simulink model "DAQsl_12lead_SZ_v3"  (R2014a)
settings: Solver=FixedStepDiscrete  StartTime=0.0  StopTime=Inf  RelTol=1e-3
undefined symbols (not defined in the file): analoginput
libraries: dspsigops x3, dspindex x3, daqlib x1
settings Model: Creator=Ssubrama  LastModifiedBy=xw8600
settings DataIOCC: MaxDataPoints=10000  SaveOutput=off  SaveTime=off
settings OptimizationCC: InitFltsAndDblsToZero=on
settings DebuggingCC: SaveWithParameterizedLinksMsg=none  UnderspecifiedInitializationDetection=Classic  SignalResolutionControl=TryResolveAllWithWarning  FcnCallInpInsideContextMsg=UseLocalSettings
settings HardwareCC: ProdBitPerLong=64  ProdBitPerPointer=64  ProdIntDivRoundTo=Zero  ProdEndianess=LittleEndian  ProdWordSize=64  ProdHWDeviceType=Intel->x86-64
settings GRTTargetCC: TargetFcnLib=ansi_tfl_tmw.mat  CombineOutputUpdateFcns=off  GRTInterface=on

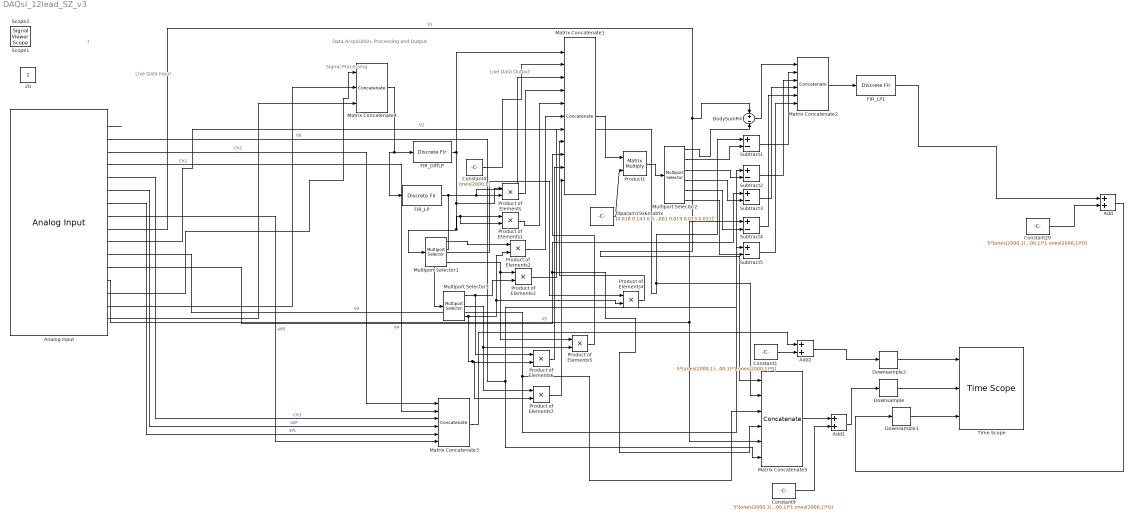
== system DAQsl_12lead_SZ_v3 ==
  note: Live Data Input
  note: Signal Processing
  note: Live Data Output
  note: ?
  note: Data Acquisition, Processing and Output
  Add : Sum
  Add1 : Sum
  Add2 : Sum
  Analog Input : daqlib/Analog Input  AcqMode=0  DeviceMenu=nidaq Dev3 (PCI-6251)  Device=nidaq Dev3 (PCI-6251)  ObjConstructor=analoginput('nidaq','Dev3')  SampleRate=48000  ActualRate=48076.9231  SamplesPerFrame=2000  InputType=SingleEnded  NChannelsSelected=16  Channels=1$0$TTL$1$#1$1$V6$1$#1$2$Ch1$1$#1$3$Ch2$1$#1$4$Ch3$1$#1$5$aVF$1$#1$6$aVL$1$#1$7$aVR$1$#1$8$V1$1$#1$9$V2$1$#1$10$V3$1$#1$11$V4$1$#1$12$V5$1$#1$13$Gx$1$#1$14$Gy$1$#1$15$Gz$1$#  NPorts=1 per hardware channel  DataType=double
      settings: SignalType=Frame-based
  BodySumR4 : Sum  Inputs=+-  SaturateOnIntegerOverflow=on  InputSameDT=on  OutDataTypeStr=Inherit: Same as first input
  Constant1 : Constant  Value=5*[ones(2000,1)*5 ones(2000,1)*4 ones(2000,1)*3 ones(2000,1)*2 ones(2000,1)*1 ones(2000,1)*0]  VectorParams1D=off
      settings: SamplingMode=Frame based
  Constant20 : Constant  Value=5*[ones(2000,1)*5 ones(2000,1)*4 ones(2000,1)*3 ones(2000,1)*2 ones(2000,1)*1 ones(2000,1)*0]  VectorParams1D=off
      settings: SamplingMode=Frame based
  Constant4 : Constant  Value=ones(2000,1)
  Constant9 : Constant  Value=5*[ones(2000,1)*5 ones(2000,1)*4 ones(2000,1)*3 ones(2000,1)*2 ones(2000,1)*1 ones(2000,1)*0]  VectorParams1D=off
      settings: SamplingMode=Frame based
  Downsample : dspsigops/Downsample  N=20  phase=0  InputProcessing=Columns as channels (frame based)  RateOptions=Enforce single-rate processing  smode=Allow multirate  fmode=Maintain input frame size  ic=0
  Downsample1 : dspsigops/Downsample  N=20  phase=0  InputProcessing=Columns as channels (frame based)  RateOptions=Enforce single-rate processing  smode=Allow multirate  fmode=Maintain input frame size  ic=0
  Downsample2 : dspsigops/Downsample  N=20  phase=0  InputProcessing=Columns as channels (frame based)  RateOptions=Enforce single-rate processing  smode=Allow multirate  fmode=Maintain input frame size  ic=0
  FIR_DiffLP : DiscreteFir  Tag=BlockMethodSubSystem  Coefficients=[-0.18062676936828148 0.075498218012372678 0.060163267428857255 0.047127582079132126 0.036106819784294142 0.02681014925394444 0.019028739148422402 0.012533880333517169 0.0071669984796646352 0.0027552314840064152 -0.00081448231664470183 -0.0036806791908466363 -0.0059307473989848453 -0.0076730993176787332 -0.0089619539864591313 -0.0098834705132522516 -0.010476162627155713 -0.010815439651932726 -0.010922412979674896 -0.010854092940204011 -0.010623964947882394 -0.010281828260079147 -0.0098295768735839738 -0.0093076194808661503 -0.0087171332221934409 -0.0080952195518808889 -0.0074299916490935501 -0.0067566400598708665 -0.0060669163247976596 -0.0053840878831306546 -0.0046956715284624667 -0.0040267199297590664 -0.0033675351882764826 -0.0027286000751785278 -0.002108607617879607 -0.0015238417303873875 -0.00094743192210984539 -0.00041768033371966662 9.7957895782735394e-05 0.00057601238716023517 0.0010248307888518354 0.0014437654277015821 0.0018365593501642741 0.0021923858617342723 0.0025292384839017273 0.0028281832383850597 0.0031059437646882987 0.0033443496347939569 0.0035673730523742425 0.003752427774854239 0.0039229917726955055 0.0040619759986883358 0.0041874782442662406 0.0042782756027622271 0.0043576942897668378 0.0044067060750872349 0.0044457562817536884 0.0044540410288122848 0.0044560643720905277 0.0044305989660153788 0.0043983184651787306 0.0043414367775261621 0.0042806358872290026 0.0041964625041126316 0.0041077120934579527 0.0039952274460846749 0.0038828867568738781 0.0037512724746293011 0.0036205033327657669 0.0034736791748717216 0.0032889244822337099 0.0032254429105413249 0.0028652076907176929 0.0029082850211105266 0.0026479711649063722 0.0023587308162685075 0.0022528173108101665 0.0021190210876191606 0.0018837093920242853 0.0016159764478156438 0.0014255307135332407 0.0012722914566817081 0.0011051792687347683 0.00087391216090881851 0.00062790988577039741 0.0003947553207023502 0.00021307525542524353 3.8419429882835532e-05 -0.00013851866134199919 -0.00035331824585213556 -0.00057153746455100574 -0.00079518720639934481 -0.00099088393330477864 -0.0011768847795266338 -0.0013366611902774078 -0.0015049172753172635 -0.0016743468203979442 -0.0018681775384048055 -0.0020506287994834366 -0.0022350623124652511 -0.0023958814720651395 -0.0025455246897644196 -0.0026681493794683125 -0.0027953157186838759 -0.0029185414486199504 -0.0030470602313935821 -0.003170822638784352 -0.0033062616061319827 -0.0034083685540330644 -0.0035137506831716507 -0.0035917717472638555 -0.0036552967807502047 -0.0037115002611477748 -0.0037592929285841514 -0.0038012849278920291 -0.0038484314440238665 -0.0038809552016502939 -0.003915923816400658 -0.0039318204175490864 -0.0039468513375555975 -0.0039355527248360334 -0.0039219335995399861 -0.0038850405920592482 -0.0038456166297130279 -0.0037875584268758089 -0.0037357892367000725 -0.0036680486958331343 -0.0036056218772497206 -0.0035256875435648108 -0.0034475962249451778 -0.0033445595331721492 -0.0032391637968775672 -0.0031120075764690808 -0.0029828631931814453 -0.0028318144386076383 -0.0026811043906390386 -0.0025110952371861922 -0.0023453505568085814 -0.002163846592305646 -0.0019895103237992234 -0.001801291958943102 -0.0016072154014195456 -0.0014196945636693326 -0.0011730884740853986 -0.00099911632268769035 -0.00073404218139398736 -0.00049829192144557055 -0.00028549369653109447 -5.506282783576677e-06 0.00024919397633001161 0.00048353320834738922 0.00072833962518251139 0.0010114071500255395 0.0012749539678287153 0.0015276715389412471 0.0017769189385540562 0.0020582940564560365 0.0023362045534717768 0.002614202508477409 0.0028710136230506861 0.0031473512240854928 0.0034284462133270521 0.0037253606974353981 0.0039994098214293505 0.0042699259854619004 0.0045289443247042843 0.0048076546226093128 0.0050751764458327117 0.0053398886724922226 0.0055788878033309307 0.0058266068769547291 0.0060625331374312072 0.0063039444342566746 0.006536104937273835 0.0067761788261536636 0.0069916195956320716 0.0071980099546128367 ...(+6580 chars)]  InputProcessing=Columns as channels (frame based)
  FIR_LP : DiscreteFir  Tag=BlockMethodSubSystem  Coefficients=[-0.016046831360515792 -0.00065949202963794772 -0.00067039658894896444 -0.000680113961541811 -0.00068755840268027585 -0.00069373348662863862 -0.00069825998158766847 -0.00070062225893785003 -0.00070116943134638197 -0.00069998300862922705 -0.00069683650818794934 -0.00069174377031850157 -0.00068465891805698231 -0.0006754671176039586 -0.00066426308006034725 -0.00065111557687173513 -0.00063595716866335708 -0.00061876858965746219 -0.00059952370199125617 -0.00057816905133744462 -0.00055474993594159874 -0.00052933462980164249 -0.00050193501018345847 -0.00047257449533386758 -0.00044127300464813848 -0.00040802895812505624 -0.00037287875518891844 -0.00033587281713210425 -0.00029703591839722911 -0.00025639926655389098 -0.00021400511216308066 -0.000169903979016367 -0.00012417368617071919 -7.6899072060668261e-05 -2.8150157008115934e-05 2.2012840404119632e-05 7.3532898375517491e-05 0.00012633250117251651 0.00018030739853822954 0.00023534639937773834 0.00029132592147520543 0.00034812020483494278 0.00040561154772518829 0.00046364631505794313 0.00052204804071215652 0.00058066809893052296 0.00063935345308781776 0.00069795947359434403 0.00075638331683252659 0.0008144673153936393 0.00087200667052411175 0.00092886523071337816 0.00098491103491506193 0.0010400300146259991 0.0010942443343466991 0.0011475182049489208 0.0011996969814079186 0.0012507656741247899 0.0013006677104798262 0.0013491930666350918 0.0013963602484677647 0.0014419368978449854 0.0014849360919130389 0.0015246732347401933 0.0015604329877536675 0.001589663683854995 0.0016110689442300034 0.0016626488924509492 0.0016801670749969633 0.0017034055881406177 0.0017242062257781157 0.001740884608416331 0.0017545721087722163 0.0017652528489535933 0.0017721296593393495 0.0017752870822966265 0.001774898562581546 0.001770787995046345 0.001762960472003177 0.0017513748993286012 0.0017357956194428426 0.0017161802261388345 0.0016926022018635637 0.0016650502257861671 0.0016335578945971853 0.0015981504382308574 0.0015587555258380591 0.0015153562862723416 0.0014680048047343904 0.00141673289877608 0.0013616004323335849 0.0013026840428024839 0.0012400261833809371 0.0011736954590057282 0.0011037979083276649 0.0010304273240276402 0.00095367644473309983 0.00087363714813433989 0.00079039072069638991 0.00070404458701325487 0.00061474337339734522 0.00052265102521284468 0.00042794153165760102 0.00033078244735946713 0.00023134271266805548 0.00012981038374990442 2.6383866326591676e-05 -7.8720638387243247e-05 -0.0001852791260239621 -0.00029309255066418093 -0.00040194826579460254 -0.00051159688026453619 -0.00062179525337211113 -0.00073228421262779182 -0.00084280009755509887 -0.00095315646127709479 -0.0010631698123428675 -0.0011725907339674574 -0.0012811859886916917 -0.0013886724649219331 -0.0014946824753083818 -0.0015989506657064674 -0.0017012114004422568 -0.0018010383222902843 -0.0018981003457104201 -0.0019921033209773596 -0.0020826208663505107 -0.0021696373876007296 -0.0022534152697132274 -0.0023336529410050173 -0.0024101808555453772 -0.0024829460735073614 -0.0025493465368724936 -0.0026056342923423959 -0.0026660896237801039 -0.0027155873088072248 -0.0027597560898392805 -0.0027992138857687344 -0.0028312885749167023 -0.0028568226553243887 -0.0028762651224427203 -0.0028887281907468195 -0.0028938572083181211 -0.0028916490204876754 -0.0028818357929839816 -0.0028643621005438689 -0.0028392507802816064 -0.0028062271598547107 -0.0027650433892605526 -0.0027155849769926309 -0.0026576966095576051 -0.0025913119936476301 -0.002516447996338678 -0.0024330280889569983 -0.002340965996042766 -0.0022402306543335519 -0.0021307704474492657 -0.0020125592717875045 -0.0018856146073182398 -0.0017499232285739519 -0.0016054780056661694 -0.0014523244548257722 -0.001290529994776534 -0.001120190883235693 -0.00094142800833800153 -0.00075434593435997482 -0.00055904539805591569 -0.00035564822940898841 -0.00014430020616271189 7.4822152403616199e-05 0.00030152760804075251 0.00053562169595984185 0.00077689558294914522 0.0010251305942399983 ...(+6591 chars)]  InputProcessing=Columns as channels (frame based)
  FIR_LP1 : DiscreteFir  Tag=BlockMethodSubSystem  Coefficients=[-0.016046831360515792 -0.00065949202963794772 -0.00067039658894896444 -0.000680113961541811 -0.00068755840268027585 -0.00069373348662863862 -0.00069825998158766847 -0.00070062225893785003 -0.00070116943134638197 -0.00069998300862922705 -0.00069683650818794934 -0.00069174377031850157 -0.00068465891805698231 -0.0006754671176039586 -0.00066426308006034725 -0.00065111557687173513 -0.00063595716866335708 -0.00061876858965746219 -0.00059952370199125617 -0.00057816905133744462 -0.00055474993594159874 -0.00052933462980164249 -0.00050193501018345847 -0.00047257449533386758 -0.00044127300464813848 -0.00040802895812505624 -0.00037287875518891844 -0.00033587281713210425 -0.00029703591839722911 -0.00025639926655389098 -0.00021400511216308066 -0.000169903979016367 -0.00012417368617071919 -7.6899072060668261e-05 -2.8150157008115934e-05 2.2012840404119632e-05 7.3532898375517491e-05 0.00012633250117251651 0.00018030739853822954 0.00023534639937773834 0.00029132592147520543 0.00034812020483494278 0.00040561154772518829 0.00046364631505794313 0.00052204804071215652 0.00058066809893052296 0.00063935345308781776 0.00069795947359434403 0.00075638331683252659 0.0008144673153936393 0.00087200667052411175 0.00092886523071337816 0.00098491103491506193 0.0010400300146259991 0.0010942443343466991 0.0011475182049489208 0.0011996969814079186 0.0012507656741247899 0.0013006677104798262 0.0013491930666350918 0.0013963602484677647 0.0014419368978449854 0.0014849360919130389 0.0015246732347401933 0.0015604329877536675 0.001589663683854995 0.0016110689442300034 0.0016626488924509492 0.0016801670749969633 0.0017034055881406177 0.0017242062257781157 0.001740884608416331 0.0017545721087722163 0.0017652528489535933 0.0017721296593393495 0.0017752870822966265 0.001774898562581546 0.001770787995046345 0.001762960472003177 0.0017513748993286012 0.0017357956194428426 0.0017161802261388345 0.0016926022018635637 0.0016650502257861671 0.0016335578945971853 0.0015981504382308574 0.0015587555258380591 0.0015153562862723416 0.0014680048047343904 0.00141673289877608 0.0013616004323335849 0.0013026840428024839 0.0012400261833809371 0.0011736954590057282 0.0011037979083276649 0.0010304273240276402 0.00095367644473309983 0.00087363714813433989 0.00079039072069638991 0.00070404458701325487 0.00061474337339734522 0.00052265102521284468 0.00042794153165760102 0.00033078244735946713 0.00023134271266805548 0.00012981038374990442 2.6383866326591676e-05 -7.8720638387243247e-05 -0.0001852791260239621 -0.00029309255066418093 -0.00040194826579460254 -0.00051159688026453619 -0.00062179525337211113 -0.00073228421262779182 -0.00084280009755509887 -0.00095315646127709479 -0.0010631698123428675 -0.0011725907339674574 -0.0012811859886916917 -0.0013886724649219331 -0.0014946824753083818 -0.0015989506657064674 -0.0017012114004422568 -0.0018010383222902843 -0.0018981003457104201 -0.0019921033209773596 -0.0020826208663505107 -0.0021696373876007296 -0.0022534152697132274 -0.0023336529410050173 -0.0024101808555453772 -0.0024829460735073614 -0.0025493465368724936 -0.0026056342923423959 -0.0026660896237801039 -0.0027155873088072248 -0.0027597560898392805 -0.0027992138857687344 -0.0028312885749167023 -0.0028568226553243887 -0.0028762651224427203 -0.0028887281907468195 -0.0028938572083181211 -0.0028916490204876754 -0.0028818357929839816 -0.0028643621005438689 -0.0028392507802816064 -0.0028062271598547107 -0.0027650433892605526 -0.0027155849769926309 -0.0026576966095576051 -0.0025913119936476301 -0.002516447996338678 -0.0024330280889569983 -0.002340965996042766 -0.0022402306543335519 -0.0021307704474492657 -0.0020125592717875045 -0.0018856146073182398 -0.0017499232285739519 -0.0016054780056661694 -0.0014523244548257722 -0.001290529994776534 -0.001120190883235693 -0.00094142800833800153 -0.00075434593435997482 -0.00055904539805591569 -0.00035564822940898841 -0.00014430020616271189 7.4822152403616199e-05 0.00030152760804075251 0.00053562169595984185 0.00077689558294914522 0.0010251305942399983 ...(+6591 chars)]  InputProcessing=Columns as channels (frame based)
  Matrix Concatenate1 : Concatenate  NumInputs=11  Mode=Multidimensional array  ConcatenateDimension=2
  Matrix Concatenate2 : Concatenate  NumInputs=6  Mode=Multidimensional array  ConcatenateDimension=2
  Matrix Concatenate3 : Concatenate  NumInputs=6  Mode=Multidimensional array  ConcatenateDimension=2
  Matrix Concatenate4 : Concatenate  NumInputs=3  Mode=Multidimensional array  ConcatenateDimension=2
  Matrix Concatenate5 : Concatenate  NumInputs=6  Mode=Multidimensional array  ConcatenateDimension=2
  Multiport Selector1 : dspindex/Multiport Selector  rowsOrCols=Columns  idxCellArray={1,2,3}  idxErrMode=Clip Index
  Multiport Selector2 : dspindex/Multiport Selector  rowsOrCols=Columns  idxCellArray={1,2,3,4,5,6}  idxErrMode=Clip Index
  Multiport Selector3 : dspindex/Multiport Selector  rowsOrCols=Columns  idxCellArray={1,2,3}  idxErrMode=Clip Index
  Product of Elements{,1..7} (8 alike) : Product
  Product1 : Product  Multiplication=Matrix(*)
  Subtract{1..5} (5 alike) : Sum  Inputs=+-
  Time Scope : TimeScope  NumInputPorts=3  DefaultConfigurationName=spbscopes.TimeScopeBlockCfg
  fitparam19x6matrix : Constant  Value=[0.018 0.143 0.006 -0.593 -0.852 0.140 -1.689 -0.045 0.038 0.008 -0.012 -0.068 0.201 -0.010 0.023 0.011 0.027 -0.032 0.038 ;0.020 0.150 0.006 -0.619 -0.887 0.140 -1.746 -0.046 0.040 0.007 -0.009 -0.068 0.210 -0.010 0.023 0.013 0.028 -0.030 0.040 ;0.019 0.262 -0.004 -0.334 -0.462 0.255 -0.843 -0.011 0.063 -0.008 0.015 -0.125 0.166 0.011 0.005 0.020 0.052 0.057 0.070 ;0.007 0.070 0.001 -0.249 -0.378 0.085 -0.628 -0.021 0.072 0.000 -0.018 -0.063 0.080 -0.009 0.006 -0.005 0.026 -0.031 0.049 ;0.006 0.185 -0.011 0.076 0.089 0.195 0.367 0.018 0.086 -0.017 -0.002 -0.096 0.020 0.013 -0.015 0.004 0.044 0.044 0.068 ;0.002 0.089 -0.009 0.080 0.080 0.097 0.423 0.015 0.045 -0.011 -0.011 -0.031 -0.004 0.006 -0.013 -0.001 0.019 0.013 0.031]'  VectorParams1D=off
  20 : Constant  IOType=siggen
  Scope1 : SignalViewerScope  IOType=viewer  NumInputPorts=3  RefreshTime=0.035000
      settings: YMin=-5~-5~-5  YMax=5~5~5
  Scope2 : SignalViewerScope  IOType=viewer  RefreshTime=0.035000
  wires:
  Analog Input/14 -> Matrix Concatenate4/1
  Matrix Concatenate4/1 -> FIR_LP/1, FIR_DiffLP/1
  Product1/1 -> Multiport Selector2/1
  fitparam19x6matrix/1 -> Product1/2
  Constant4/1 -> Matrix Concatenate1/2
  FIR_LP/1 -> Product of Elements/2, Matrix Concatenate1/3, Multiport Selector3/1
  Multiport Selector2/1 -> BodySumR4/2
  FIR_DiffLP/1 -> Matrix Concatenate1/1, Product of Elements/1, Multiport Selector1/1, Product of Elements1/1, Product of Elements1/2
  Matrix Concatenate1/1 -> Product1/1
  Analog Input/9 -> Matrix Concatenate5/1, BodySumR4/1  "V1"
  Analog Input/10 -> Subtract1/1, Matrix Concatenate5/2  "V2"
  Analog Input/11 -> Matrix Concatenate5/3, Subtract2/1  "V3"
  Analog Input/12 -> Matrix Concatenate5/4, Subtract3/1  "V4"
  Analog Input/2 -> Matrix Concatenate5/6, Subtract5/1  "V6"
  Analog Input/13 -> Subtract4/1, Matrix Concatenate5/5  "V5"
  BodySumR4/1 -> Matrix Concatenate2/1
  Multiport Selector2/2 -> Subtract1/2
  Subtract1/1 -> Matrix Concatenate2/2
  Multiport Selector2/3 -> Subtract2/2
  Multiport Selector2/4 -> Subtract3/2
  Multiport Selector2/5 -> Subtract4/2
  Multiport Selector2/6 -> Subtract5/2
  Subtract2/1 -> Matrix Concatenate2/3
  Subtract3/1 -> Matrix Concatenate2/4
  Subtract4/1 -> Matrix Concatenate2/5
  Subtract5/1 -> Matrix Concatenate2/6
  Matrix Concatenate2/1 -> FIR_LP1/1
  FIR_LP1/1 -> Add/1
  Matrix Concatenate3/1 -> Add2/1
  Constant20/1 -> Add/2
  Add/1 -> Downsample1/1
  Matrix Concatenate5/1 -> Add1/1
  Constant9/1 -> Add1/2
  Add1/1 -> Downsample/1
  Downsample/1 -> Time Scope/2
  Downsample1/1 -> Time Scope/3
  Downsample2/1 -> Time Scope/1
  Analog Input/3 -> Matrix Concatenate3/1  "Ch1"
  Analog Input/4 -> Matrix Concatenate3/2  "Ch2"
  Analog Input/5 -> Matrix Concatenate3/3  "Ch3"
  Analog Input/6 -> Matrix Concatenate3/4  "aVF"
  Analog Input/7 -> Matrix Concatenate3/5  "aVL"
  Analog Input/8 -> Matrix Concatenate3/6  "aVR"
  Analog Input/1 -> ?
  Add2/1 -> Downsample2/1
  Constant1/1 -> Add2/2
  Analog Input/15 -> Matrix Concatenate4/2
  Analog Input/16 -> Matrix Concatenate4/3
  Product of Elements/1 -> Matrix Concatenate1/4
  Product of Elements1/1 -> Matrix Concatenate1/5
  Multiport Selector1/1 -> Product of Elements2/1
  Multiport Selector3/3 -> Product of Elements7/2, Product of Elements6/2, Product of Elements4/2, Product of Elements2/2
  Product of Elements2/1 -> Matrix Concatenate1/6
  Multiport Selector1/3 -> Product of Elements5/1, Product of Elements3/1
  Multiport Selector3/1 -> Product of Elements6/1, Product of Elements3/2
  Product of Elements3/1 -> Matrix Concatenate1/7
  Multiport Selector1/2 -> Product of Elements4/1
  Product of Elements4/1 -> Matrix Concatenate1/8
  Multiport Selector3/2 -> Product of Elements7/1, Product of Elements5/2
  Product of Elements5/1 -> Matrix Concatenate1/9
  Product of Elements7/1 -> Matrix Concatenate1/11
  Product of Elements6/1 -> Matrix Concatenate1/10
